simulink model "xEMU_SimulationModel3_rule1"  (R2017b)
settings: Solver=ode4  StartTime=0.0  StopTime=8192  FixedStep=0.01  RelTol=1e-3
undefined symbols (not defined in the file): a1, a2, a3, a4, ACO, BAT, Battery, DCT, DRT, EMS, ENV, Fahrzyklus_VS_modell, height_BAT, leistung, lib_bat, Maximum, Maximum_position, Num_cells, P_FC_max_long, P_FC_min_long, P_FC_step_max, Pbat_charge_max, Pbat_discharge_max, Pfc_max, Pfc_min, SOC_tar, time_peaks, TRM, velocity_peaks
libraries: simulink x5
(part 1 of 15)
settings Model: SimulationMode=accelerator  Creator=tne  LastModifiedBy=chenzhu1
settings SolverCC: ZeroCrossAlgorithm=Adaptive
settings OptimizationCC: EfficientMapNaN2IntZero=off
settings HardwareCC: TargetBitPerLong=64  TargetBitPerPointer=64  TargetBitPerSizeT=64  TargetBitPerPtrDiffT=64  TargetLongLongMode=on  TargetIntDivRoundTo=Zero  TargetEndianess=LittleEndian  TargetWordSize=64  TargetHWDeviceType=MATLAB Host  ProdEqTarget=off
settings CodeAppCC: MaxIdLength=128
settings GRTTargetCC: TargetLangStandard=C89/C90 (ANSI)  CombineOutputUpdateFcns=off  GRTInterface=on

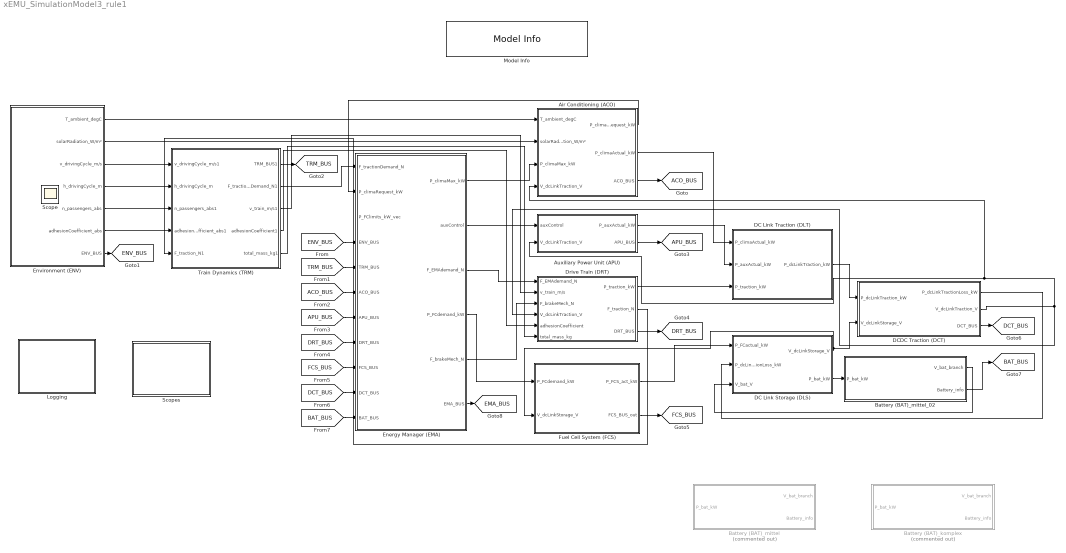
== system xEMU_SimulationModel3_rule1 ==
  Air Conditioning (ACO) : Subsystem
  Auxiliary Power Unit (APU) : Subsystem
  Battery (BAT)_komplex : Subsystem  Commented=on  AncestorBlock=lib_bat/Battery (BAT)  mask{n_series=BAT.model.n_series, n_parallel=BAT.model.n_parallel, Temp=BAT.model.Temp, SoC=BAT.model.SoC, Rser=BAT.model.Rser, R1=BAT.model.R1, Tau1=BAT.model.Tau1, R2=BAT.model.R2, Tau2=BAT.model.Tau2, Phi2=BAT.model.Phi2, R3=BAT.model.R3, Tau3=BAT.model.Tau3, Phi3=BAT.model.Phi3, R4=BAT.model.R4, Tau4=BAT.model.Tau4, R5=BAT.model.R5, Tau5=BAT.model.Tau5, Sigma2=BAT.model.Sigma2, CLim2=BAT.model.CLim2, Sigma3=BAT.model.Sigma3, CLim3=BAT.model.CLim3, ROCV=BAT.model.ROCV, UOCV=BAT.model.UOCV, OCV2=BAT.model.OCV2, SOC2=BAT.model.SOC2, TEMP2=BAT.model.TEMP2}
  Battery (BAT)_mittel : Subsystem  Commented=on  AncestorBlock=lib_bat/Battery (BAT)  mask{n_series=BAT.model.n_series, n_parallel=BAT.model.n_parallel, Temp=BAT.model.Temp, SoC=BAT.model.SoC, Rser=BAT.model.Rser, R1=BAT.model.R1, Tau1=BAT.model.Tau1, R2=BAT.model.R2, Tau2=BAT.model.Tau2, Phi2=BAT.model.Phi2, R3=BAT.model.R3, Tau3=BAT.model.Tau3, Phi3=BAT.model.Phi3, R4=BAT.model.R4, Tau4=BAT.model.Tau4, R5=BAT.model.R5, Tau5=BAT.model.Tau5, Sigma2=BAT.model.Sigma2, CLim2=BAT.model.CLim2, Sigma3=BAT.model.Sigma3, CLim3=BAT.model.CLim3, ROCV=BAT.model.ROCV, UOCV=BAT.model.UOCV, OCV2=BAT.model.OCV2, SOC2=BAT.model.SOC2, TEMP2=BAT.model.TEMP2}
  Battery (BAT)_mittel_02 : Subsystem  AncestorBlock=lib_bat/Battery (BAT)  mask{n_series=BAT.model.n_series, n_parallel=BAT.model.n_parallel, Temp=BAT.model.Temp, SoC=BAT.model.SoC, Rser=BAT.model.Rser, R1=BAT.model.R1, Tau1=BAT.model.Tau1, R2=BAT.model.R2, Tau2=BAT.model.Tau2, Phi2=BAT.model.Phi2, R3=BAT.model.R3, Tau3=BAT.model.Tau3, Phi3=BAT.model.Phi3, R4=BAT.model.R4, Tau4=BAT.model.Tau4, R5=BAT.model.R5, Tau5=BAT.model.Tau5, Sigma2=BAT.model.Sigma2, CLim2=BAT.model.CLim2, Sigma3=BAT.model.Sigma3, CLim3=BAT.model.CLim3, ROCV=BAT.model.ROCV, UOCV=BAT.model.UOCV, OCV2=BAT.model.OCV2, SOC2=BAT.model.SOC2, TEMP2=BAT.model.TEMP2}
  DC Link Storage (DLS) : Subsystem
  DC Link Traction (DLT) : Subsystem
  DCDC Traction (DCT) : Subsystem  AncestorBlock=lib_dct/DCDC Traction (DCT)  mask{fs_DCDC_Hz=DCT.fs_DCDC_Hz}
  Drive Train (DRT) : Subsystem  AncestorBlock=lib_drt/Drive Train (DRT)  mask{gearratio_drt=DRT.motor.gearratio_drt, R_wheel_drt_m=DRT.slipmodel.R_wheel_drt_m, g_drt=DRT.slipmodel.g_drt, fr_drt_abs=DRT.slipmodel.fr_drt_abs, J_drt=DRT.slipmodel.J_drt, Schub_drt=DRT.slipmodel.Schub_drt, a_drt=DRT.slipmodel.a_drt, b_drt=DRT.slipmodel.b_drt, C11_drt=DRT.slipmodel.C11_drt, speedvector=DRT.motor.speedvector, torquevector=DRT.motor.torquevector, eta=DRT.motor.eta, cosphi=DRT.motor.cosphi, I_strang=DRT.motor.I_strang, U_LL=DRT.motor.U_LL, Pv_motor=DRT.motor.Pv_motor, torque_untergrenze=DRT.motor.torque_untergrenze, torque_obergrenze=DRT.motor.torque_obergrenze, torquevector2=DRT.motor.torquevector2, speedvector2=DRT.motor.speedvector2, cosphi2=DRT.motor.cosphi2, Pv_untergrenze=DRT.motor.Pv_untergrenze, Pv_obergrenze=DRT.motor.Pv_obergrenze, U_LL_untergrenze=DRT.motor.U_LL_untergrenze, U_LL_obergrenze=DRT.motor.U_LL_obergrenze, I_strang_untergrenze=DRT.motor.I_strang_untergrenze, cosphi_obergrenze=DRT.motor.cosphi_obergrenze, cosphi_untergrenze=DRT.motor.cosphi_untergrenze, I_strang_obergrenze=DRT.motor.I_strang_obergrenze}
  Energy Manager (EMA) : Subsystem  AncestorBlock=lib_ems/Energy Manager (EMA)
  Environment (ENV) : Subsystem
  Fuel Cell System (FCS) : Subsystem  AncestorBlock=lib_fcs/Fuel Cell System (FCS)
  Logging : Subsystem
  Model Info : simulink/Model-Wide Utilities/Model Info  Frame=on  DisplayStringWithTags=|  HorizontalTextAlignment=Center  LeftAlignmentValue=0.5
      | Model name: %<ModelName>
      | Created: %<Created>
      | Model version:%<ModelVersion>
      | Last modified by: hp
      | Last modification date: %<LastModificationDate>
  Scopes : Subsystem
  Train Dynamics (TRM) : Subsystem  AncestorBlock=lib_trm/Train Dynamics (TDN)1  mask{m_train_tdn_kg=TRM.m_train_tdn_kg, Cw_tdn_abs=TRM.Cw_tdn_abs, A_tdn_m2=TRM.A_tdn_m2, e_tdn_abs=TRM.e_tdn_abs, PI_tdn=TRM.PI_tdn, m_passenger_tdn_kg=TRM.m_passenger_tdn_kg, g_drt=TRM.g_drt, gearratio_drt=DRT.motor.gearratio_drt, R_wheel_drt_m=DRT.slipmodel.R_wheel_drt_m, speedvector=DRT.motor.speedvector, torquevector=DRT.motor.torquevector, torque_untergrenze=DRT.motor.torque_untergrenze, torque_obergrenze=DRT.motor.torque_obergrenze}
  Scope : Scope
  tag scope: ACO_BUS=global, APU_BUS=global, BAT_BUS=global, DCT_BUS=global, DRT_BUS=global, EMA_BUS=global, ENV_BUS=global, FCS_BUS=global, TRM_BUS=global
  wires:
  Environment (ENV)/1(T_ambient_degC) -> Air Conditioning (ACO)/1(T_ambient_degC)
  Environment (ENV)/2(solarRadiation_W/m²) -> Air Conditioning (ACO)/2(solarRadiation_W/m²)
  Air Conditioning (ACO)/2(P_climaActual_kW) -> DC Link Traction (DLT)/1(P_climaActual_kW)
  Auxiliary Power Unit (APU)/1(P_auxActual_kW) -> DC Link Traction (DLT)/2(P_auxActual_kW)
  Environment (ENV)/7(ENV_BUS) -> [ENV_BUS]
  DC Link Storage (DLS)/1(V_dcLinkStorage_V) -> DCDC Traction (DCT)/2(V_dcLinkStorage_V), Fuel Cell System (FCS)/2(V_dcLinkStorage_V)
  DC Link Traction (DLT)/1(P_dcLinkTraction_kW) -> DCDC Traction (DCT)/1(P_dcLinkTraction_kW)
  DCDC Traction (DCT)/1(P_dcLinkTractionLoss_kW) -> DC Link Storage (DLS)/2(P_dcLinkTractionLoss_kW)
  Drive Train (DRT)/1(P_traction_kW) -> DC Link Traction (DLT)/3(P_traction_kW)
  Drive Train (DRT)/2(F_traction_N) -> Train Dynamics (TRM)/5(F_traction_N1)
  Environment (ENV)/4(h_drivingCycle_m) -> Train Dynamics (TRM)/2(h_drivingCycle_m)
  Train Dynamics (TRM)/3(v_train_m/s1) -> Drive Train (DRT)/2(v_train_m/s)
  Train Dynamics (TRM)/4(adhesionCoefficient1) -> Drive Train (DRT)/5("adhesionCoefficient ")
  Train Dynamics (TRM)/5(total_mass_kg1) -> Drive Train (DRT)/6(total_mass_kg)
  Air Conditioning (ACO)/1(P_climaRequest_kW) -> Energy Manager (EMA)/2("P_climaRequest_kW ")
  Energy Manager (EMA)/4(P_FCdemand_kW) -> Fuel Cell System (FCS)/1(P_FCdemand_kW)
  Energy Manager (EMA)/5(F_brakeMech_N) -> Drive Train (DRT)/3(F_brakeMech_N)
  Energy Manager (EMA)/6(EMA_BUS) -> [EMA_BUS]
  [TRM_BUS] -> Energy Manager (EMA)/5(TRM_BUS)
  [ACO_BUS] -> Energy Manager (EMA)/6(ACO_BUS)
  [APU_BUS] -> Energy Manager (EMA)/7(APU_BUS)
  [DRT_BUS] -> Energy Manager (EMA)/8(DRT_BUS)
  [FCS_BUS] -> Energy Manager (EMA)/9(FCS_BUS)
  [DCT_BUS] -> Energy Manager (EMA)/10(DCT_BUS)
  [BAT_BUS] -> Energy Manager (EMA)/11(BAT_BUS)
  [ENV_BUS] -> Energy Manager (EMA)/4(ENV_BUS)
  Energy Manager (EMA)/3(F_EMAdemand_N) -> Drive Train (DRT)/1(F_EMAdemand_N)
  Energy Manager (EMA)/2(auxControl) -> Auxiliary Power Unit (APU)/1(auxControl)
  Energy Manager (EMA)/1(P_climaMax_kW) -> Air Conditioning (ACO)/3(P_climaMax_kW)
  DCDC Traction (DCT)/2(V_dcLinkTraction_V) -> Drive Train (DRT)/4(V_dcLinkTraction_V), Auxiliary Power Unit (APU)/2(V_dcLinkTraction_V), Air Conditioning (ACO)/4(V_dcLinkTraction_V)
  DCDC Traction (DCT)/3(DCT_BUS) -> [DCT_BUS]
  Drive Train (DRT)/3(DRT_BUS) -> [DRT_BUS]
  Auxiliary Power Unit (APU)/2(APU_BUS) -> [APU_BUS]
  Air Conditioning (ACO)/3(ACO_BUS) -> [ACO_BUS]
  Environment (ENV)/3(v_drivingCycle_m/s) -> Train Dynamics (TRM)/1(v_drivingCycle_m/s1)
  Environment (ENV)/5(n_passengers_abs) -> Train Dynamics (TRM)/3(n_passengers_abs1)
  Environment (ENV)/6(adhesionCoefficient_abs) -> Train Dynamics (TRM)/4(adhesionCoefficient_abs1)
  Train Dynamics (TRM)/1(TRM_BUS1) -> [TRM_BUS]
  Train Dynamics (TRM)/2(F_tractionDemand_N1) -> Energy Manager (EMA)/1(F_tractionDemand_N)
  Fuel Cell System (FCS)/1(P_FCS_act_kW) -> DC Link Storage (DLS)/1(P_FCactual_kW)
  Fuel Cell System (FCS)/2(FCS_BUS_out) -> [FCS_BUS]
  DC Link Storage (DLS)/2(P_bat_kW) -> Battery (BAT)_mittel_02/1(P_bat_kW)
  Battery (BAT)_mittel_02/1(V_bat_branch) -> DC Link Storage (DLS)/3(V_bat_V)
  Battery (BAT)_mittel_02/2(Battery_info) -> [BAT_BUS]

== system xEMU_SimulationModel3_rule1/Air Conditioning (ACO) ==
  T_ambient_degC : Inport
  solarRadiation_W/m² : Inport  Port=2
  P_climaMax_kW : Inport  Port=3
  V_dcLinkTraction_V : Inport  Port=4
  Bus Creator1 : BusCreator  Inputs=3
  Constant : Constant
  Constant1 : Constant
  Divide : Product  Inputs=*/
  Divide1 : Product  Inputs=*/
  Gain : Gain  Gain=ACO.Awin/2
  Gain1 : Gain  Gain=ACO.Awall
  Gain2 : Gain  Gain=ACO.Awin
  Gain3 : Gain  Gain=116.3
  Heat gain : Fcn  Expr=u^2/ACO.R_warm
  Subtract : Sum
  Subtract1 : Sum  Inputs=+++++
  Sum : Sum  Inputs=-+|
  Tsoll : Constant  Value=25
  Unit Delay : UnitDelay  SampleTime=-1
  Wall-Conduct-Convection-Coefficient : Fcn  Expr=1/ACO.a1+ACO.s1/ACO.lambda1+ACO.s2/ACO.lambda2+ACO.s3/ACO.lambda3+1/u
  "Window-Conduct-Convection-Coeffcient " : Fcn  Expr=1/ACO.a1+ACO.swin/ACO.lambdawin+1/u
  approximation from passenger to ventilation : Gain  Gain=5/3
  efficient : Gain  Gain=1/3
  exterior coefficient : Fcn  Expr=9+3.5*u^0.66
  w-kw : Gain  Gain=1/1000
  P_climaRequest_kW : Outport
  P_climaActual_kW : Outport  Port=2
  ACO_BUS : Outport  Port=3
  wires:
  Unit Delay/1 -> ACO_BUS/1
  Gain/1 -> Subtract1/2  "Radiation"
  T_ambient_degC/1 -> Sum/2
  Tsoll/1 -> Sum/1
  Sum/1 -> Divide1/1, Divide/1
  "Window-Conduct-Convection-Coeffcient "/1 -> Divide1/2
  Wall-Conduct-Convection-Coefficient/1 -> Divide/2
  Divide/1 -> Gain1/1
  Divide1/1 -> Gain2/1
  Gain1/1 -> Subtract/1
  Gain2/1 -> Subtract/2
  Subtract/1 -> Subtract1/1  "Conduction&Convection"
  exterior coefficient/1 -> "Window-Conduct-Convection-Coeffcient "/1, Wall-Conduct-Convection-Coefficient/1
  [v_ist] -> exterior coefficient/1
  Gain3/1 -> approximation from passenger to ventilation/1, Subtract1/3  "passengers'load"
  approximation from passenger to ventilation/1 -> Subtract1/4  "ventilation"
  Subtract1/1 -> w-kw/1
  efficient/1 -> P_climaActual_kW/1, P_climaRequest_kW/1
  V_dcLinkTraction_V/1 -> Heat gain/1
  Heat gain/1 -> Subtract1/5
  w-kw/1 -> efficient/1
  Bus Creator1/1 -> Unit Delay/1
  Constant1/1 -> Bus Creator1/2  "signal2"
  Constant/1 -> Bus Creator1/1  "signal1"
  P_climaMax_kW/1 -> Bus Creator1/3  "P_Klima"
  solarRadiation_W/m²/1 -> Gain/1
  [n_passengers] -> Gain3/1

== system xEMU_SimulationModel3_rule1/Auxiliary Power Unit (APU) ==
  auxControl : Inport
  V_dcLinkTraction_V : Inport  Port=2
  Constant : Constant  Value=30
  Unit Delay : UnitDelay  SampleTime=-1
  P_auxActual_kW : Outport
  APU_BUS : Outport  Port=2
  wires:
  Constant/1 -> Unit Delay/1
  Unit Delay/1 -> APU_BUS/1, P_auxActual_kW/1  "P_aux"

== system xEMU_SimulationModel3_rule1/Battery (BAT)_komplex ==
  P_bat_kW : Inport
  Bus Creator : BusCreator  Inputs=12
  Delay : Delay  DelayLength=1
  Display1 : Display
  Divide : Product  Inputs=*/
  Gain : Gain  Gain=-1
  Gain1 : Gain  Gain=1/100
  Gain2 : Gain  Gain=-1
  Integrator1 : Integrator  LimitOutput=on  LowerSaturationLimit=0
  MATLAB Function : MATLAB Function  TreatAsAtomicUnit=on
  Scope : Scope
  Scope6 : Scope
  Subsystem : Subsystem
  cell2pack : Gain  Gain=370
  kW->W : Gain  Gain=1000
  pack2cell : Gain  Gain=1/9
  V_bat_branch : Outport
  Battery_info : Outport  Port=2
  wires:
  Bus Creator/1 -> Battery_info/1
  kW->W/1 -> Divide/1
  Delay/1 -> Gain2/1, MATLAB Function/2(I_bat), pack2cell/1  "I_bat"
  P_bat_kW/1 -> Bus Creator/5, Gain/1  "P_bat"
  Divide/1 -> Delay/1  "I_Pack_A"
  cell2pack/1 -> V_bat_branch/1, Bus Creator/1, Display1/1, Divide/2  "V_bat"
  pack2cell/1 -> Subsystem/1(In2)  "I_Cell_A"
  Subsystem/1(CellVoltage) -> cell2pack/1
  Subsystem/5(SoC_Percent) -> Gain1/1, Bus Creator/8  "SOC"
  Gain/1 -> kW->W/1  "P_bat"
  MATLAB Function/1(Battery_consume_eff_rate) -> Integrator1/1
  Gain1/1 -> Scope6/1, MATLAB Function/1(SOC_i)
  Integrator1/1 -> Scope/1
  Gain2/1 -> Bus Creator/2  "I_bat"
  [T_CellElement1] -> MATLAB Function/3(Temp)

== system xEMU_SimulationModel3_rule1/Battery (BAT)_mittel ==
  note: I positive --> Charge
  note: I negative --> Discharge
  P_bat_kW : Inport
  Battery : Subsystem
  Bus : BusCreator  Inputs=6
  Bus Creator1 : BusCreator  Inputs=12
  Bus Selector : BusSelector  OutputSignals=soc.signal1
  Delay : Delay  DelayLength=1
  Display1 : Display
  Divide : Product  Inputs=*/
  Gain : Gain  Gain=-1
  Gain1 : Gain  Gain=-1
  Scope : Scope
  Scope1 : Scope
  Subsystem1 : Subsystem  Commented=on
  To Workspace : ToWorkspace  VariableName=Batt_temp_1s1p_thevenin  SaveFormat=Structure With Time  SampleTime=-1
  cell2pack : Gain  Gain=370
  cell2pack1 : Gain
  kW->W : Gain  Gain=1000
  pack2cell : Gain  Gain=1/9
  V_bat_branch : Outport
  Battery_info : Outport  Port=2
  wires:
  kW->W/1 -> Divide/1
  Delay/1 -> Gain1/1, pack2cell/1
  P_bat_kW/1 -> Gain/1, Bus Creator1/5  "P_bat"
  Divide/1 -> Delay/1  "I_Pack_A"
  cell2pack/1 -> V_bat_branch/1, Display1/1, Divide/2, Bus Creator1/1  "V_bat"
  pack2cell/1 -> Battery/1(I_Bat_source[A])  "I_Cell_A"
  Battery/3(CellVoltage) -> Bus/3, cell2pack/1, Scope1/1
  Gain/1 -> kW->W/1
  Battery/6(SoC_[0..1]) -> Bus/6
  Battery/2(CellPower) -> Bus/2
  Battery/5(CellTemp) -> To Workspace/1, Scope/1, Bus/5
  Battery/4(CellVoltage1) -> Bus/4
  Battery/1(SoC_Percent) -> Bus/1  "soc"
  Bus/1 -> Bus Selector/1
  Bus Selector/1 -> cell2pack1/1  "<signal1>"
  Bus Creator1/1 -> Battery_info/1
  cell2pack1/1 -> Bus Creator1/8  "SOC"
  Gain1/1 -> Bus Creator1/9  "I_bat"

== system xEMU_SimulationModel3_rule1/Battery (BAT)_mittel_02 ==
  note: I positive --> Charge
  note: I negative --> Discharge
  P_bat_kW : Inport
  " " : Gain
  Bus : BusCreator  Inputs=6
  Bus Creator1 : BusCreator  Inputs=12
  Bus Selector : BusSelector  OutputSignals=soc
  Cell : Subsystem
  Cell_temperatur : Scope
  Delay : Delay  DelayLength=1
  Display1 : Display
  Divide : Product  Inputs=*/
  Gain : Gain  Gain=-1
  Gain1 : Gain  Gain=-1
  Scope1 : Scope
  Soc in % : Display
  To Workspace : ToWorkspace  VariableName=Batt_temp_1s1p_thevenin  SaveFormat=Structure With Time  SampleTime=-1
  cell2pack : Gain  Gain=370
  cell_voltage : Display
  kW->W : Gain  Gain=1000
  pack2cell : Gain  Gain=1/9
  V_bat_branch : Outport
  Battery_info : Outport  Port=2
  wires:
  kW->W/1 -> Divide/1
  Delay/1 -> Gain1/1, pack2cell/1
  P_bat_kW/1 -> Gain/1, Bus Creator1/5  "P_bat"
  Divide/1 -> Delay/1  "I_Pack_A"
  cell2pack/1 -> V_bat_branch/1, Display1/1, Divide/2, Bus Creator1/1  "V_bat"
  pack2cell/1 -> Cell/1(ExcitationCurrent)  "I_Cell_A"
  Cell/5(TotalVoltage) -> cell2pack/1, Scope1/1, Bus/3, cell_voltage/1  "cell_voltage"
  Gain/1 -> kW->W/1
  Cell/9(TemperatureVector) -> Bus/6, Cell_temperatur/1, To Workspace/1  "cell_temperature"
  Cell/6(TotalCurrent) -> Bus/4  "cell_current"
  Cell/4(SocVector) -> Soc in %/1, Bus/1  "soc"
  Bus Selector/1 -> " "/1  "<soc>"
  Bus Creator1/1 -> Battery_info/1
  " "/1 -> Bus Creator1/8  "SOC"
  Gain1/1 -> Bus Creator1/9  "I_bat"
  Cell/2(CurrentVector) -> ?
  Bus/1 -> Bus Selector/1
  Cell/7(TotalHeatGeneration) -> Bus/5  "cell_heat"

== system xEMU_SimulationModel3_rule1/DC Link Storage (DLS) ==
  note: die Summe aller Leistung und Verluste
  note: die Versorgung aus FC
  note: die Versorgung aus Battery
  P_FCactual_kW : Inport
  P_dcLinkTractionLoss_kW : Inport  Port=2
  V_bat_V : Inport  Port=3
  Constant : Constant
  Integrator1 : Integrator
  Integrator2 : Integrator
  MATLAB Function : MATLAB Function  TreatAsAtomicUnit=on
  Subtract : Sum  Inputs=-+
  V_dcLinkStorage_V : Outport
  P_bat_kW : Outport  Port=2
  tag scope: P_Demand=global
  wires:
  V_bat_V/1 -> Integrator2/1, V_dcLinkStorage_V/1
  Subtract/1 -> P_bat_kW/1
  P_FCactual_kW/1 -> Subtract/1
  P_dcLinkTractionLoss_kW/1 -> [P_Demand], Subtract/2
  Constant/1 -> Integrator1/1
  Integrator1/1 -> MATLAB Function/1(t)
  Integrator2/1 -> MATLAB Function/2(v_bat_total)
  MATLAB Function/1(v_bat_average) -> ?

== system xEMU_SimulationModel3_rule1/DC Link Traction (DLT) ==
  P_climaActual_kW : Inport
  P_auxActual_kW : Inport  Port=2
  P_traction_kW : Inport  Port=3
  Sum : Sum  Inputs=|+++
  P_dcLinkTraction_kW : Outport
  wires:
  P_auxActual_kW/1 -> Sum/2
  P_climaActual_kW/1 -> Sum/1
  P_traction_kW/1 -> Sum/3
  Sum/1 -> P_dcLinkTraction_kW/1

== system xEMU_SimulationModel3_rule1/DCDC Traction (DCT) ==
  P_dcLinkTraction_kW : Inport
  V_dcLinkStorage_V : Inport  Port=2
  DCDC_elektrisch_Modellierung : Subsystem
  DCDC_thermische_Modellirung : Subsystem
  P_dcLinkTractionLoss_kW : Outport
  V_dcLinkTraction_V : Outport  Port=2
  DCT_BUS : Outport  Port=3
  wires:
  P_dcLinkTraction_kW/1 -> DCDC_elektrisch_Modellierung/1(P_load_vor_dcdc_converter1)  "P_load_vor_dcdc_converter"
  V_dcLinkStorage_V/1 -> DCDC_elektrisch_Modellierung/2(V_dcLinkStorage_V1)
  DCDC_elektrisch_Modellierung/1(V_dcLinkTraction_V) -> V_dcLinkTraction_V/1
  DCDC_elektrisch_Modellierung/4("IGBT_Pv_kW ") -> DCDC_thermische_Modellirung/2(igbt_loss_kW)
  DCDC_elektrisch_Modellierung/2("DCT_BUS ") -> DCT_BUS/1
  DCDC_elektrisch_Modellierung/5(Diode_Pv_kW) -> DCDC_thermische_Modellirung/1(Diode_loss_kW)
  DCDC_thermische_Modellirung/1(IGBT_Temp_Celsius) -> DCDC_elektrisch_Modellierung/4(IGBT _Junction_Temp1)
  DCDC_thermische_Modellirung/2(Diode_Temp_Celsius) -> DCDC_elektrisch_Modellierung/3(Diode _Junction_Temp1)
  DCDC_elektrisch_Modellierung/3(P_dcLinkTractionLoad_kW) -> P_dcLinkTractionLoss_kW/1

== system xEMU_SimulationModel3_rule1/Drive Train (DRT) ==
  F_EMAdemand_N : Inport
  v_train_m/s : Inport  Port=2
  F_brakeMech_N : Inport  Port=3
  V_dcLinkTraction_V : Inport  Port=4
  "adhesionCoefficient " : Inport  Port=5
  total_mass_kg : Inport  Port=6
  Aufteilung rad-undmotormomente : Subsystem
  Bus Creator : BusCreator  Inputs=5
  Converter and traction motor : Subsystem
  Gain : Gain  Gain=gearratio_drt
  Mechanical Brake : Subsystem
  Product{,1..4} (5 alike) : Product
  "Slipmodel and Traction " : Subsystem
  Subtract : Sum
  Sum : Sum  Inputs=++|
  Unit Delay : UnitDelay  SampleTime=-1
  gear efficiency : MATLAB Function  TreatAsAtomicUnit=on
  gear_efficiency : Constant  Value=DRT.motor.gear_efficiency_drt
  P_traction_kW : Outport
  F_traction_N : Outport  Port=2
  DRT_BUS : Outport  Port=3
  wires:
  Unit Delay/1 -> DRT_BUS/1
  V_dcLinkTraction_V/1 -> Converter and traction motor/3(v_dc)
  F_EMAdemand_N/1 -> Aufteilung rad-undmotormomente/1(F_EMAdemand_N)
  Mechanical Brake/1(Out1) -> Sum/1
  Product/1 -> P_traction_kW/1  "P_motor_elekrisch+Pacdc"
  Converter and traction motor/1("T_singelmotor_Nm ") -> Gain/1  "m"
  Aufteilung rad-undmotormomente/4(T_brake_axis_Nm) -> Mechanical Brake/1(In1)
  Gain/1 -> gear efficiency/1(t_motor)
  Aufteilung rad-undmotormomente/1(T_demandperdrive_Nm) -> Converter and traction motor/1(T_demand)
  Aufteilung rad-undmotormomente/2(n_motor_rpm) -> Converter and traction motor/2(n), Bus Creator/5  "n_motor_rpm"
  F_brakeMech_N/1 -> Aufteilung rad-undmotormomente/2(F_brake_N)
  Converter and traction motor/2("Pel_singlemotor_kW ") -> Product/2
  "Slipmodel and Traction "/2(WheelSpeed_rad/s) -> Aufteilung rad-undmotormomente/3("WheelSpeed_rad/s ")
  Sum/1 -> "Slipmodel and Traction "/1(T_EMAdemandper_axis_Nm)
  "adhesionCoefficient "/1 -> "Slipmodel and Traction "/3(adhesionCoefficient_abs)
  total_mass_kg/1 -> "Slipmodel and Traction "/4(total mass_kg)
  v_train_m/s/1 -> "Slipmodel and Traction "/2(v_train_m/s)
  Bus Creator/1 -> Unit Delay/1
  "Slipmodel and Traction "/1(F_traction_peraxis_N) -> Product2/2
  Product2/1 -> F_traction_N/1
  Product3/1 -> Bus Creator/2  "P_motor_mechanisch"
  Aufteilung rad-undmotormomente/3(Number_drives_available) -> Product/1, Product1/1, Product4/1, Product3/1, Product2/1, "Slipmodel and Traction "/5(numberdrivesavailable)
  [P_motor_mechanic] -> Product3/2  "P_motor_mechanic"
  [Pv_motor] -> Product4/2
  Product4/1 -> Subtract/2, Bus Creator/3  "P_motor_Verlust"
  Product1/1 -> Subtract/1, Bus Creator/1  "P_acdc_Verlust"
  Subtract/1 -> Bus Creator/4  "P_motor_Verlust+Pacdc"
  [Pv_ACDC] -> Product1/2  "P_acdc_Verlust"
  gear efficiency/1(t_axis) -> Sum/2
  gear_efficiency/1 -> gear efficiency/2(data)

== system xEMU_SimulationModel3_rule1/Energy Manager (EMA) ==
  F_tractionDemand_N : Inport
  "P_climaRequest_kW " : Inport  Port=2
  P_FClimits_kW_vec : Inport  Port=3
  ENV_BUS : Inport  Port=4
  TRM_BUS : Inport  Port=5
  ACO_BUS : Inport  Port=6
  APU_BUS : Inport  Port=7
  DRT_BUS : Inport  Port=8
  FCS_BUS : Inport  Port=9
  DCT_BUS : Inport  Port=10
  BAT_BUS : Inport  Port=11
  Berechnung der available Traktionsleitung : Subsystem
  Bus Creator1 : BusCreator  Inputs=8
  Bus Selector : BusSelector  OutputSignals=v_drivingCycle_m/s,Steigung%
  Bus Selector1 : BusSelector  OutputSignals=v_train_m/s
  Bus Selector2 : BusSelector  OutputSignals=P_motor_Verlust+Pacdc,n_motor_rpm
  Bus Selector3 : BusSelector  OutputSignals=P_dcdc_Verlust,P_dcLinkTractionLoad
  Bus Selector4 : BusSelector  OutputSignals=SOC,V_bat
  Demux : Demux
  Display{,1..3} (4 alike) : Display
  Kern von EMS : Subsystem
  Scope : Scope
  Umrechnung von Kraft zu Leistung : Subsystem
  Umrechnung von Leistung auf Kraft : Subsystem
  Umrechnung von Leistung auf Kraft2 : Subsystem
  P_climaMax_kW : Outport
  auxControl : Outport  Port=2
  F_EMAdemand_N : Outport  Port=3
  P_FCdemand_kW : Outport  Port=4
  F_brakeMech_N : Outport  Port=5
  EMA_BUS : Outport  Port=6
  tag scope: F_EMAdemand_N=global, P_apu=global, P_clima=global, n_motor_rpm=global, v_soll=global
  wires:
  Bus Selector/1 -> Kern von EMS/2(<v_train_m/s>_soll), [v_soll]  "<v_drivingCycle_m/s>"
  Bus Selector1/1 -> Umrechnung von Kraft zu Leistung/2(<v_train_m/s>), Umrechnung von Leistung auf Kraft2/3(<v_train_m/s>), Umrechnung von Leistung auf Kraft/3(<v_drivingCycle_m/s>)  "<v_train_m/s>"
  Kern von EMS/1(P_FCdemand_kW) -> P_FCdemand_kW/1, Bus Creator1/6  "P_Fc_demand"
  [mode] -> Bus Creator1/7  "mode"
  [P_apu] -> Bus Creator1/4  "P_apu"
  [P_clima] -> Bus Creator1/3  "P_clima"
  Bus Selector3/1 -> Berechnung der available Traktionsleitung/3(<P_dcdc_Verlust>), Umrechnung von Kraft zu Leistung/4(<P_dcdc_Verlust>)  "<P_dcdc_Verlust>"
  Bus Selector2/1 -> Berechnung der available Traktionsleitung/2(<P_motor_Verlust+Pacdc>), Umrechnung von Kraft zu Leistung/3(<P_motor_Verlust+Pacdc>)  "<P_motor_Verlust+Pacdc>"
  Bus Creator1/1 -> EMA_BUS/1
  Bus Selector4/2 -> Kern von EMS/4(<V_bat_V>)  "<V_bat>"
  Bus Selector4/1 -> Kern von EMS/3(<SOC_perc>)  "<SOC>"
  APU_BUS/1 -> [P_apu]
  ENV_BUS/1 -> Bus Selector/1
  TRM_BUS/1 -> Bus Selector1/1
  DRT_BUS/1 -> Bus Selector2/1
  BAT_BUS/1 -> Bus Selector4/1
  "P_climaRequest_kW "/1 -> P_climaMax_kW/1, [P_clima]
  DCT_BUS/1 -> Bus Selector3/1
  P_FClimits_kW_vec/1 -> Demux/1
  Bus Selector2/2 -> [n_motor_rpm]  "<n_motor_rpm>"
  Umrechnung von Kraft zu Leistung/2(P_drive_demand) -> Umrechnung von Leistung auf Kraft/2(P_drive_demand), Bus Creator1/1
  F_tractionDemand_N/1 -> Umrechnung von Kraft zu Leistung/1(F_tractionDemand_N)
  Umrechnung von Kraft zu Leistung/1(P_load_wunsch) -> Display/1, Kern von EMS/1(P_load_wunsch_kw)
  Kern von EMS/2(P_load_available) -> Display1/1, Scope/1, Berechnung der available Traktionsleitung/1(P_load_available)
  Berechnung der available Traktionsleitung/1(P_traction_available) -> Display2/1, Umrechnung von Leistung auf Kraft/1(P_traction_available)
  Umrechnung von Leistung auf Kraft2/3(F_EMAdemand_N) -> Display3/1, [F_EMAdemand_N], F_EMAdemand_N/1
  Umrechnung von Leistung auf Kraft/1(F_brakeMech_N) -> Umrechnung von Leistung auf Kraft2/1(F_brakeMech_N1)
  Umrechnung von Leistung auf Kraft/2(F_EMAdemand_N) -> Umrechnung von Leistung auf Kraft2/2(F_EMAdemand_N1)
  Umrechnung von Leistung auf Kraft2/1(F_available_nach_EMA) -> Bus Creator1/8
  Umrechnung von Leistung auf Kraft2/2(F_brakeMech_N) -> F_brakeMech_N/1

== system xEMU_SimulationModel3_rule1/Environment (ENV) ==
  %-1 : Gain  Gain=1/100
  1-D Lookup Table : Lookup_n-D  NumberOfTableDimensions=1  BreakpointsForDimension1=ENV.height.position  Table=ENV.height.Height  InternalRulePriority=Speed  RndMeth=Simplest  InputSameDT=on
  Bus Creator : BusCreator  Inputs=2
  Fahrzyklus : simulink/Sources/Repeating Sequence  rep_seq_t=ENV.fahrzyklus.time  rep_seq_y=ENV.fahrzyklus.v
  Integrator : Integrator
  Integrator1 : Integrator
  Scope1 : Scope
  Steigung : Lookup_n-D  NumberOfTableDimensions=1  BreakpointsForDimension1=ENV.steigung.position  Table=ENV.steigung.Steigung  InternalRulePriority=Speed  RndMeth=Simplest  InputSameDT=on
  T_ambient : Constant  Value=ENV.temperatur
  adhesionCoefficient : Constant  Value=ENV.adhesionCoefficient
  number of Passengers : Constant  Value=ENV.number_passengers
  solarRadiation : Constant  Value=ENV.solarRadiation
  T_ambient_degC : Outport
  solarRadiation_W/m² : Outport  Port=2
  v_drivingCycle_m/s : Outport  Port=3
  h_drivingCycle_m : Outport  Port=4
  n_passengers_abs : Outport  Port=5
  adhesionCoefficient_abs : Outport  Port=6
  ENV_BUS : Outport  Port=7
  tag scope: n_passengers=global
  wires:
  Bus Creator/1 -> ENV_BUS/1
  Fahrzyklus/1 -> v_drivingCycle_m/s/1, Bus Creator/1, Integrator1/1  "v_drivingCycle_m/s"
  Steigung/1 -> Integrator/1, Bus Creator/2, %-1/1  "Steigung%"
  adhesionCoefficient/1 -> adhesionCoefficient_abs/1
  T_ambient/1 -> T_ambient_degC/1
  solarRadiation/1 -> solarRadiation_W/m²/1
  Integrator1/1 -> 1-D Lookup Table/1, Steigung/1
  %-1/1 -> Scope1/1, h_drivingCycle_m/1
  number of Passengers/1 -> [n_passengers], n_passengers_abs/1
  Integrator/1 -> ?

== system xEMU_SimulationModel3_rule1/Fuel Cell System (FCS) ==
  P_FCdemand_kW : Inport
  V_dcLinkStorage_V : Inport  Port=2
  "FC_DCDC " : Subsystem  AncestorBlock=lib_fcs/Fuel Cell System (FCS)/FC_controller
  "FC_controller " : Subsystem
  FC_system : Subsystem  AncestorBlock=lib_fcs/Fuel Cell System (FCS)/FC_controller
  Unit Delay : UnitDelay  SampleTime=-1
  P_FCS_act_kW : Outport
  FCS_BUS_out : Outport  Port=2
  wires:
  Unit Delay/1 -> FCS_BUS_out/1
  FC_system/1(FCS_state_BUS) -> "FC_controller "/3(FC_state_BUS)
  "FC_DCDC "/1(P_DCDC_act_kW) -> P_FCS_act_kW/1, "FC_controller "/5(p_fc_act)
  FC_system/3(i_act_fcs) -> "FC_DCDC "/4(i_act_fcs)
  "FC_DCDC "/2(i_demand_dcdc_fc) -> FC_system/2(i_demand_dcdc_fc)
  "FC_controller "/2(i_demand) -> "FC_DCDC "/1(i_demand_ext)
  FC_system/2(V_FCS) -> "FC_DCDC "/3(V_FCS), "FC_controller "/4(V_FCS)
  "FC_controller "/1(FCS_BUS) -> Unit Delay/1
  V_dcLinkStorage_V/1 -> "FC_controller "/2(V_dcLink), "FC_DCDC "/2(V_dcLink)
  P_FCdemand_kW/1 -> FC_system/1("P_fc "), "FC_controller "/1(p_demand_ext)

== system xEMU_SimulationModel3_rule1/Logging ==
  To Workspace : ToWorkspace  VariableName=bat_bus  SaveFormat=Timeseries  SampleTime=-1
  wires:
  [BAT_BUS] -> To Workspace/1

== system xEMU_SimulationModel3_rule1/Scopes ==
  Battery Scope : Subsystem
  Energy Manager Scope : Subsystem
  "Fuel cell Scope " : Subsystem
  Train Dynamics&Environment Scope : Subsystem

== system xEMU_SimulationModel3_rule1/Train Dynamics (TRM) ==
  v_drivingCycle_m/s1 : Inport
  h_drivingCycle_m : Inport  Port=2
  n_passengers_abs1 : Inport  Port=3
  adhesionCoefficient_abs1 : Inport  Port=4
  F_traction_N1 : Inport  Port=5
  Variant Subsystem : Subsystem  Variant=on  OverrideUsingVariant=Variant
  TRM_BUS1 : Outport
  F_tractionDemand_N1 : Outport  Port=2
  v_train_m/s1 : Outport  Port=3
  adhesionCoefficient1 : Outport  Port=4
  total_mass_kg1 : Outport  Port=5
  tag scope: total_mass=global, v_ist=global
  wires:
  Variant Subsystem/2(F_tractionDemand_N) -> F_tractionDemand_N1/1  "F_tractionDemand_N"
  Variant Subsystem/3(v_train_m/s) -> [v_ist], v_train_m/s1/1  "v_train_m/s"
  F_traction_N1/1 -> Variant Subsystem/5(F_traction_N)
  adhesionCoefficient_abs1/1 -> Variant Subsystem/4(adhesionCoefficient_abs)
  n_passengers_abs1/1 -> Variant Subsystem/3(n_passengers_abs)
  h_drivingCycle_m/1 -> Variant Subsystem/2(h_drivingCycle_m)
  Variant Subsystem/1(TRM_BUS) -> TRM_BUS1/1
  Variant Subsystem/4(adhesionCoefficient) -> adhesionCoefficient1/1
  Variant Subsystem/5(total_mass_kg) -> [total_mass], total_mass_kg1/1
  v_drivingCycle_m/s1/1 -> Variant Subsystem/1(v_drivingCycle_m/s)

== system xEMU_SimulationModel3_rule1/Battery (BAT)_komplex/Subsystem ==
  In2 : Inport
  ActiveBalancing : Subsystem
  ActiveBalancingCellCurrents : Constant  Value=[0]
  CellCurrentMatrices : Subsystem
  CellCurrents : Subsystem
  CellPowerValues : Subsystem
  CellVoltageMatrices : Subsystem
  Demux : Demux  Outputs=2
  ElectricalCircuit : Subsystem
  MatrixAxC : Subsystem
  MatrixX_alg : Subsystem
  PowerMatrix : Subsystem
  SystemStates : Subsystem
  Thermal : Subsystem
  CellVoltage : Outport
  CellPower : Outport  Port=2
  CellTemp : Outport  Port=3
  CellVoltage1 : Outport  Port=4
  SoC_Percent : Outport  Port=5
  tag scope: InputCurrent=global
  wires:
  ActiveBalancingCellCurrents/1 -> ActiveBalancing/1(CellCurrents)
  PowerMatrix/1(Components) -> CellPowerValues/1(CellPower)
  CellPowerValues/1(Out1) -> CellPower/1
  Thermal/1(Out1) -> CellTemp/1  "CellTemperature"
  Demux/2 -> CellVoltage1/1
  Demux/1 -> CellVoltage/1  "Cell_Voltage"
  CellCurrentMatrices/1(Components) -> CellCurrents/1(CellCurrents)
  In2/1 -> [InputCurrent]
  ElectricalCircuit/1(Out1) -> SoC_Percent/1
  CellVoltageMatrices/1(Components) -> Demux/1

== system xEMU_SimulationModel3_rule1/Battery (BAT)_mittel/Battery ==
  I_Bat_source[A] : Inport
  'ID3_ObjR : GotoTagVisibility  GotoTag=ID3_ObjR
  'ID3_ObjTau : GotoTagVisibility  GotoTag=ID3_ObjTau
  'ID4_ObjR : GotoTagVisibility  GotoTag=ID4_ObjR
  'ID4_ObjTau : GotoTagVisibility  GotoTag=ID4_ObjTau
  'ID5_ObjR : GotoTagVisibility  GotoTag=ID5_ObjR
  'ID5_ObjTau : GotoTagVisibility  GotoTag=ID5_ObjTau
  'State1 : GotoTagVisibility  GotoTag=State1
  'State2 : GotoTagVisibility  GotoTag=State2
  'State3 : GotoTagVisibility  GotoTag=State3
  'T_CellElement1 : GotoTagVisibility  GotoTag=T_CellElement1
  ActBal1 : GotoTagVisibility  GotoTag=ActBal1
  ActiveBalancing : Subsystem
  ActiveBalancingCellCurrents : Constant  Value=[0]
  BalancerBus_goto : GotoTagVisibility  GotoTag=BalancerBus
  CellCurrentMatrices : Subsystem
  CellCurrents : Subsystem
  CellPowerValues : Subsystem
  CellVoltageMatrices : Subsystem
  Demux : Demux  Outputs=2
  ElectricalCircuit : Subsystem
  ID2_ObjR : GotoTagVisibility  GotoTag=ID2_ObjR
  ID6_ObjV : GotoTagVisibility  GotoTag=ID6_ObjV
  I_CellElement_goto1 : GotoTagVisibility  GotoTag=I_CellElement1
  InputCurrent_goto : GotoTagVisibility  GotoTag=InputCurrent
  MatrixAxC : Subsystem
  MatrixX_alg : Subsystem
  P_CellElement_goto1 : GotoTagVisibility  GotoTag=P_CellElement1
  PowerMatrix : Subsystem
  SOC_fraction : Gain  Gain=0.01
  StatesBus_goto : GotoTagVisibility  GotoTag=StatesBus
  SystemStates : Subsystem
  Thermal : Subsystem
  SoC_Percent : Outport
  CellPower : Outport  Port=2
  CellVoltage : Outport  Port=3
  CellVoltage1 : Outport  Port=4
  CellTemp : Outport  Port=5
  SoC_[0..1] : Outport  Port=6
  tag scope: InputCurrent=scoped
  wires:
  Thermal/1(CellTemp_Bus) -> CellTemp/1
  ActiveBalancingCellCurrents/1 -> ActiveBalancing/1(CellCurrents)
  CellCurrentMatrices/1(Components) -> CellCurrents/1(CellCurrents)
  CellPowerValues/1(Out1) -> CellPower/1
  CellVoltageMatrices/1(Components) -> Demux/1
  PowerMatrix/1(Components) -> CellPowerValues/1(CellPower)
  I_Bat_source[A]/1 -> [InputCurrent]
  Demux/2 -> CellVoltage1/1
  Demux/1 -> CellVoltage/1
  SOC_fraction/1 -> SoC_[0..1]/1
  ElectricalCircuit/1(SoC_%_Bus) -> SoC_Percent/1, SOC_fraction/1

== system xEMU_SimulationModel3_rule1/Battery (BAT)_mittel/Subsystem1 ==
  In2 : Inport
  ActiveBalancing : Subsystem
  ActiveBalancingCellCurrents : Constant  Value=[0]
  CellCurrentMatrices : Subsystem
  CellCurrents : Subsystem
  CellPowerValues : Subsystem
  CellVoltageMatrices : Subsystem
  Demux : Demux  Outputs=2
  ElectricalCircuit : Subsystem
  MatrixAxC : Subsystem
  MatrixX_alg : Subsystem
  PowerMatrix : Subsystem
  SystemStates : Subsystem
  Thermal : Subsystem
  CellVoltage : Outport
  CellPower : Outport  Port=2
  CellTemp : Outport  Port=3
  CellVoltage1 : Outport  Port=4
  SoC_Percent : Outport  Port=5
  tag scope: InputCurrent=global
  wires:
  ActiveBalancingCellCurrents/1 -> ActiveBalancing/1(CellCurrents)
  PowerMatrix/1(Components) -> CellPowerValues/1(CellPower)
  CellPowerValues/1(Out1) -> CellPower/1
  Thermal/1(Out1) -> CellTemp/1  "CellTemperature"
  Demux/2 -> CellVoltage1/1
  Demux/1 -> CellVoltage/1  "Cell_Voltage"
  CellCurrentMatrices/1(Components) -> CellCurrents/1(CellCurrents)
  In2/1 -> [InputCurrent]
  ElectricalCircuit/1(Out1) -> SoC_Percent/1
  CellVoltageMatrices/1(Components) -> Demux/1

== system xEMU_SimulationModel3_rule1/Battery (BAT)_mittel_02/Cell ==
  ExcitationCurrent : Inport
  BalancingCurrent : Inport  Port=2
  AmbientTemperature : Inport  Port=3
  Reset : Inport  Port=4
  ActiveBalancing : Subsystem
  CellCurrentMatrices : Subsystem
  CellCurrents : Subsystem
  CellPowerValues : Subsystem
  CellVoltageMatrices : Subsystem
  ElectricalCircuit : Subsystem
  MatrixAxC : Subsystem
  MatrixX_alg : Subsystem
  NumCellElements : Constant
  PowerMatrix : Subsystem
  SoC_Vector : Subsystem
  SystemStates : Subsystem
  Temperature_Vector : Subsystem
  Thermal : Subsystem
  TotalValues : Subsystem
  VoltageVector : Outport
  CurrentVector : Outport  Port=2
  OhmicHeatGenerationVector : Outport  Port=3
  SocVector : Outport  Port=4
  TotalVoltage : Outport  Port=5
  TotalCurrent : Outport  Port=6
  TotalHeatGeneration : Outport  Port=7
  NumberOfBatteries : Outport  Port=8
  TemperatureVector : Outport  Port=9
  ProbeTemperatureVector : Outport  Port=10
  tag scope: AirTemperature=global, InputCurrent=global, Reset=global
  wires:
  Temperature_Vector/1(TemperatureVector) -> TemperatureVector/1
  BalancingCurrent/1 -> ActiveBalancing/1(CellCurrents)
  TotalValues/1(Current) -> TotalCurrent/1
  CellCurrentMatrices/1(Components) -> CellCurrents/1(CellCurrents), CurrentVector/1
  PowerMatrix/1(Components) -> OhmicHeatGenerationVector/1, CellPowerValues/1(CellPower)
  TotalValues/3(Power) -> TotalHeatGeneration/1
  TotalValues/2(Voltage) -> TotalVoltage/1
  SoC_Vector/1(SocVector) -> SocVector/1
  Reset/1 -> [Reset]
  [ThermalProbeTemperatures] -> ProbeTemperatureVector/1
  ExcitationCurrent/1 -> [InputCurrent]
  NumCellElements/1 -> NumberOfBatteries/1
  CellVoltageMatrices/1(Components) -> VoltageVector/1
  AmbientTemperature/1 -> [AirTemperature]

== system xEMU_SimulationModel3_rule1/DCDC Traction (DCT)/DCDC_elektrisch_Modellierung ==
  note: schaltverlust diode
  note: diodeverlust
  note: gesamte verluste
      | in DCDC wandler
  note: igbtverlust
  P_load_vor_dcdc_converter1 : Inport
  V_dcLinkStorage_V1 : Inport  Port=2
  Diode _Junction_Temp1 : Inport  Port=3
  IGBT _Junction_Temp1 : Inport  Port=4
  Add5 : Sum  Inputs=+++
  Add6 : Sum
  Bus Creator1 : BusCreator  Inputs=3
  Delay : Delay  DelayLength=1
  Delay1 : Delay  DelayLength=1
  Divide2 : Product  Inputs=*/
  Efficiency measurment : Subsystem
  Efficiency measurment1 : Subsystem
  Efficiency1 : Display
  Efficiency2 : Display
  Gain{1,7..9} (4 alike) : Gain  Gain=1 / 1000
  Gain2 : Gain  Gain=1 / 6
  Gain3 : Gain  Gain=1 / 6
  Gain6 : Gain  Gain=1000
  Unit Delay1 : UnitDelay  SampleTime=-1
  Zwischenkreisspanung1 : Constant  Value=DCT.dc_dink_voltage
  n-D Lookup Diode : Lookup_n-D  NumberOfTableDimensions=4  BreakpointsForDimension1=DCT.loss_diode.D1_U_B  BreakpointsForDimension2=DCT.loss_diode.D2_U_DC  BreakpointsForDimension3=DCT.loss_diode.D3_I_DC  BreakpointsForDimension4=DCT.loss_diode.D4_T_jun  Table=DCT.loss_diode.loss  InternalRulePriority=Speed  RndMeth=Simplest  InputSameDT=on
  n-D Lookup IGBT : Lookup_n-D  NumberOfTableDimensions=4  BreakpointsForDimension1=DCT.loss_igbt.D1_U_B  BreakpointsForDimension2=DCT.loss_igbt.D2_U_DC  BreakpointsForDimension3=DCT.loss_igbt.D3_I_DC  BreakpointsForDimension4=DCT.loss_igbt.D4_T_jun  Table=DCT.loss_igbt.loss  InternalRulePriority=Speed  RndMeth=Simplest  InputSameDT=on
  n-D Lookup Inductor : Lookup_n-D  NumberOfTableDimensions=4  BreakpointsForDimension1=DCT.loss_inductor.D1_U_B  BreakpointsForDimension2=DCT.loss_inductor.D2_U_DC  BreakpointsForDimension3=DCT.loss_inductor.D3_I_DC  BreakpointsForDimension4=DCT.loss_inductor.D4_T_jun  Table=DCT.loss_inductor.loss  InternalRulePriority=Speed  RndMeth=Simplest  InputSameDT=on
  V_dcLinkTraction_V : Outport
  "DCT_BUS " : Outport  Port=2
  P_dcLinkTractionLoad_kW : Outport  Port=3
  "IGBT_Pv_kW " : Outport  Port=4
  Diode_Pv_kW : Outport  Port=5
  tag scope: Loss_Inductor=global
  wires:
  Gain8/1 -> Delay1/1
  V_dcLinkStorage_V1/1 -> n-D Lookup IGBT/1, n-D Lookup Diode/1, n-D Lookup Inductor/1
  Gain6/1 -> Divide2/1
  Divide2/1 -> n-D Lookup Diode/3, n-D Lookup Inductor/3, n-D Lookup IGBT/3
  Gain7/1 -> Efficiency measurment1/2(In2), Bus Creator1/1, Add6/2  "P_dcdc_Verlust"
  Add5/1 -> Gain7/1
  Bus Creator1/1 -> Unit Delay1/1
  Add6/1 -> P_dcLinkTractionLoad_kW/1, Efficiency measurment/2(In2), Bus Creator1/2  "P_dcLinkTractionLoad"
  n-D Lookup IGBT/1 -> Gain2/1, Add5/1
  Diode _Junction_Temp1/1 -> n-D Lookup Inductor/4, n-D Lookup IGBT/4
  Unit Delay1/1 -> "DCT_BUS "/1
  Gain9/1 -> Delay/1
  IGBT _Junction_Temp1/1 -> n-D Lookup Diode/4
  n-D Lookup Diode/1 -> Add5/2, Gain3/1
  Zwischenkreisspanung1/1 -> V_dcLinkTraction_V/1, n-D Lookup Diode/2, Divide2/2, n-D Lookup Inductor/2, n-D Lookup IGBT/2
  n-D Lookup Inductor/1 -> Gain1/1
  Gain1/1 -> [Loss_Inductor], Add5/3
  Gain2/1 -> Gain8/1
  Gain3/1 -> Gain9/1
  Efficiency measurment1/1(Efficiency) -> Efficiency2/1
  Efficiency measurment/1(Efficiency) -> Efficiency1/1
  P_load_vor_dcdc_converter1/1 -> Efficiency measurment/1(In1), Efficiency measurment1/1(In1), Add6/1, Bus Creator1/3, Gain6/1  "P_load_vor_dcdc_converter"
  Delay1/1 -> "IGBT_Pv_kW "/1
  Delay/1 -> Diode_Pv_kW/1

== system xEMU_SimulationModel3_rule1/DCDC Traction (DCT)/DCDC_thermische_Modellirung ==
  Diode_loss_kW : Inport
  igbt_loss_kW : Inport  Port=2
  "Heat sink Temperatur " : Constant  Value=DCT.thermal.heatsink_temperatur
  "Heat sink_Temperatur " : Constant  Value=DCT.thermal.heatsink_temperatur
  R_c_s_module_diode_side : Gain  Gain=DCT.thermal.R_c_s_module_diode_side
  R_c_s_module_igbt_side : Gain  Gain=DCT.thermal.R_c_s_module_igbt_side
  R_j_c_diode : Gain  Gain=DCT.thermal.R_j_c_diode
  R_j_c_igbt : Gain  Gain=DCT.thermal.R_j_c_igbt
  Sum : Sum  Inputs=|+++
  Sum1 : Sum  Inputs=|+++
  IGBT_Temp_Celsius : Outport
  Diode_Temp_Celsius : Outport  Port=2
  wires:
  igbt_loss_kW/1 -> R_j_c_igbt/1, R_c_s_module_igbt_side/1
  Diode_loss_kW/1 -> R_j_c_diode/1, R_c_s_module_diode_side/1
  "Heat sink Temperatur "/1 -> Sum/1
  "Heat sink_Temperatur "/1 -> Sum1/3
  R_j_c_diode/1 -> Sum1/2
  R_j_c_igbt/1 -> Sum/2
  R_c_s_module_igbt_side/1 -> Sum/3
  R_c_s_module_diode_side/1 -> Sum1/1
  Sum/1 -> IGBT_Temp_Celsius/1
  Sum1/1 -> Diode_Temp_Celsius/1

== system xEMU_SimulationModel3_rule1/Drive Train (DRT)/Aufteilung rad-undmotormomente ==
  F_EMAdemand_N : Inport
  F_brake_N : Inport  Port=2
  "WheelSpeed_rad/s " : Inport  Port=3
  Constant : Constant  Value=3
  Divide1 : Product  Inputs=*/
  Divide2 : Product  Inputs=/*
  Gain : Gain  Gain=gearratio_drt*60/2/pi
  Gain1 : Gain  Gain=R_wheel_drt_m/gearratio_drt
  Gain2 : Gain  Gain=R_wheel_drt_m
  T_demandperdrive_Nm : Outport
  n_motor_rpm : Outport  Port=2
  Number_drives_available : Outport  Port=3
  T_brake_axis_Nm : Outport  Port=4
  tag scope: num_EM=global
  wires:
  F_brake_N/1 -> Gain2/1
  Gain/1 -> n_motor_rpm/1
  Gain1/1 -> Divide1/1
  Constant/1 -> [num_EM], Divide2/1, Divide1/2, Number_drives_available/1
  Divide1/1 -> T_demandperdrive_Nm/1
  "WheelSpeed_rad/s "/1 -> Gain/1
  Gain2/1 -> Divide2/2
  Divide2/1 -> T_brake_axis_Nm/1
  F_EMAdemand_N/1 -> Gain1/1

== system xEMU_SimulationModel3_rule1/Drive Train (DRT)/Converter and traction motor ==
  T_demand : Inport
  n : Inport  Port=2
  v_dc : Inport  Port=3
  Converter_DRT : Subsystem
  Efficiency measument2 : Display
  Efficiency measurment1 : Subsystem
  Efficiency2 : Display
  Gain : Gain  Gain=2*pi/60
  Multiply : Product
  P_el : Display
  P_mech : Display
  Sum : Sum  Inputs=|++
  traction_motor_kennfeldbasiert : Subsystem
  "T_singelmotor_Nm " : Outport
  "Pel_singlemotor_kW " : Outport  Port=2
  tag scope: P_motor=global, Pv_ACDC=global, Pv_motor=global
  wires:
  Converter_DRT/2(Efficiency_out) -> Efficiency measument2/1
  traction_motor_kennfeldbasiert/1(P_el) -> P_el/1, [P_motor], Efficiency measurment1/1(In1), Sum/1
  v_dc/1 -> Converter_DRT/2(V_dcLinkStorage_V)
  Multiply/1 -> Gain/1
  Sum/1 -> "Pel_singlemotor_kW "/1
  n/1 -> Multiply/2, Converter_DRT/5(RPM), traction_motor_kennfeldbasiert/2(n)
  traction_motor_kennfeldbasiert/4(I_1) -> Converter_DRT/1("I_traction_motor ")
  traction_motor_kennfeldbasiert/2(M_ist) -> "T_singelmotor_Nm "/1
  Efficiency measurment1/1(Efficiency) -> Efficiency2/1
  traction_motor_kennfeldbasiert/3(U_1) -> Converter_DRT/3(V_Drive_V)
  traction_motor_kennfeldbasiert/6(Pv_motor) -> [Pv_motor]
  traction_motor_kennfeldbasiert/5(cos_phi) -> Converter_DRT/4(Cos_Phi_Phaseshift)
  T_demand/1 -> Multiply/1, traction_motor_kennfeldbasiert/1(M_soll)
  Converter_DRT/1(P_dcLinkTractionLoss_kW) -> Sum/2, Efficiency measurment1/2(In2), [Pv_ACDC]
  Gain/1 -> P_mech/1

== system xEMU_SimulationModel3_rule1/Drive Train (DRT)/Mechanical Brake ==
  In1 : Inport
  Out1 : Outport
  wires:
  In1/1 -> Out1/1

== system xEMU_SimulationModel3_rule1/Drive Train (DRT)/Slipmodel and Traction  ==
  T_EMAdemandper_axis_Nm : Inport
  v_train_m/s : Inport  Port=2
  adhesionCoefficient_abs : Inport  Port=3
  total mass_kg : Inport  Port=4
  numberdrivesavailable : Inport  Port=5
  "Tire Resistance " : Subsystem
  Variant Subsystem1 : Subsystem  Variant=on  OverrideUsingVariant=Variant2
  F_traction_peraxis_N : Outport
  WheelSpeed_rad/s : Outport  Port=2
  wires:
  "Tire Resistance "/1(resistance of tire) -> Variant Subsystem1/4(Resistance of tire)
  total mass_kg/1 -> "Tire Resistance "/2(total mass_kg)
  numberdrivesavailable/1 -> "Tire Resistance "/1(numberdrivesavailable)
  T_EMAdemandper_axis_Nm/1 -> Variant Subsystem1/1(T_EMAdemandper_axis_Nm)
  v_train_m/s/1 -> Variant Subsystem1/2(v_train_m/s)
  adhesionCoefficient_abs/1 -> Variant Subsystem1/3(adhesionCoefficient_abs)
  "Tire Resistance "/2(Fz_tire) -> Variant Subsystem1/5(Fz_tire)
  Variant Subsystem1/3(f_traction_tire) -> "Tire Resistance "/3(f_traction_tire)
  Variant Subsystem1/1(F_traction_peraxis_N) -> F_traction_peraxis_N/1
  Variant Subsystem1/2(WheelSpeed_rad/s) -> WheelSpeed_rad/s/1

== system xEMU_SimulationModel3_rule1/Energy Manager (EMA)/Berechnung der available Traktionsleitung ==
  P_load_available : Inport
  <P_motor_Verlust+Pacdc> : Inport  Port=2
  <P_dcdc_Verlust> : Inport  Port=3
  Subtract1 : Sum  Inputs=+-
  Subtract2 : Sum  Inputs=-+-
  Subtract3 : Sum  Inputs=+-
  eta_getriebe 1 : Gain
  P_traction_available : Outport
  wires:
  <P_dcdc_Verlust>/1 -> Subtract1/2
  <P_motor_Verlust+Pacdc>/1 -> Subtract3/2
  eta_getriebe 1/1 -> P_traction_available/1
  [P_clima] -> Subtract2/1
  [P_apu] -> Subtract2/3
  P_load_available/1 -> Subtract1/1
  Subtract3/1 -> eta_getriebe 1/1
  Subtract2/1 -> Subtract3/1
  Subtract1/1 -> Subtract2/2

== system xEMU_SimulationModel3_rule1/Energy Manager (EMA)/Kern von EMS ==
  note: P_load_wunsch_kw
  note: P_fc_kann
  P_load_wunsch_kw : Inport
  <v_train_m/s>_soll : Inport  Port=2
  <SOC_perc> : Inport  Port=3
  <V_bat_V> : Inport  Port=4
  Add : Sum
  Gain3 : Gain  Gain=1/100
  "Leistungsflussverteilug " : Subsystem
  P_load_aver : Subsystem
  Rate Limiter : RateLimiter  RisingSlewLimit=EMS.Fuelcell.P_fc_anstieg_max  FallingSlewLimit=EMS.Fuelcell.P_fc_abstieg_max  SampleTimeMode=inherited
  Saturation : Saturate  UpperLimit=EMS.Bat.power_discharge_max+EMS.Fuelcell.P_fc_max  LowerLimit=-EMS.Bat.power_charge_max + EMS.pload_average
  Saturation1 : Saturate  UpperLimit=EMS.Fuelcell.P_fc_max  LowerLimit=EMS.Fuelcell.P_fc_min
  Scope{1..4} (4 alike) : Scope
  Subsystem : Subsystem
  P_FCdemand_kW : Outport
  P_load_available : Outport  Port=2
  wires:
  <SOC_perc>/1 -> Gain3/1
  P_load_wunsch_kw/1 -> Saturation/1
  <v_train_m/s>_soll/1 -> P_load_aver/1(V_SOLL)
  Saturation/1 -> "Leistungsflussverteilug "/1(P_load), Subsystem/1(P_load_wunsch_kw), Scope2/1
  Gain3/1 -> P_load_aver/2(SOC), "Leistungsflussverteilug "/3(SoC), Subsystem/3(SOC)
  Add/1 -> P_load_available/1
  <V_bat_V>/1 -> Subsystem/4(<V_bat_V>)
  Subsystem/1(P_bat_kann) -> Add/2
  P_load_aver/1(P_load_mean) -> Scope3/1, "Leistungsflussverteilug "/2("P_load_aver ")
  Rate Limiter/1 -> Scope4/1, P_FCdemand_kW/1, Subsystem/2(P_fc_kann), Add/1
  Saturation1/1 -> Rate Limiter/1
  "Leistungsflussverteilug "/1(P_FCdemand_kW) -> Scope1/1, Saturation1/1

== system xEMU_SimulationModel3_rule1/Energy Manager (EMA)/Umrechnung von Kraft zu Leistung ==
  F_tractionDemand_N : Inport
  <v_train_m/s> : Inport  Port=2
  <P_motor_Verlust+Pacdc> : Inport  Port=3
  <P_dcdc_Verlust> : Inport  Port=4
  Constant2 : Constant  Value=10^-5
  Gain : Gain  Gain=1/ 1000
  Gain1 : Gain  Gain=1/ 1000
  Leistung nach ACDC : Sum
  Leistungsbedarf der Energiequelle : Sum
  Min2 : MinMax  Function=max  Inputs=2
  Product : Product
  Product1 : Product
  Sum1 : Sum  Inputs=|++
  "eta_getriebe " : Gain
  power into inverter1 : Sum  Inputs=+++
  P_load_wunsch : Outport
  P_drive_demand : Outport  Port=2
  tag scope: F_demand=global, F_driver=global
  wires:
  [F_EMA_min] -> Min2/2
  Min2/1 -> Product/1, [F_demand]
  Product/1 -> Gain/1
  Gain1/1 -> P_drive_demand/1  "P_drive_demand"
  Product1/1 -> Gain1/1
  F_tractionDemand_N/1 -> [F_driver], Product1/1, Min2/1
  "eta_getriebe "/1 -> Leistung nach ACDC/1  "P_drive_demand"
  Constant2/1 -> Sum1/2
  Sum1/1 -> Product/2
  Gain/1 -> "eta_getriebe "/1
  [P_apu] -> power into inverter1/3
  Leistungsbedarf der Energiequelle/1 -> P_load_wunsch/1  "P_load_wunsch"
  [P_clima] -> power into inverter1/2
  power into inverter1/1 -> Leistungsbedarf der Energiequelle/1
  Leistung nach ACDC/1 -> power into inverter1/1
  <P_motor_Verlust+Pacdc>/1 -> Leistung nach ACDC/2
  <P_dcdc_Verlust>/1 -> Leistungsbedarf der Energiequelle/2
  <v_train_m/s>/1 -> Sum1/1, Product1/2

== system xEMU_SimulationModel3_rule1/Energy Manager (EMA)/Umrechnung von Leistung auf Kraft ==
  P_traction_available : Inport
  P_drive_demand : Inport  Port=2
  <v_drivingCycle_m/s> : Inport  Port=3
  Constant3 : Constant  Value=10^-5
  Divide3 : Product  Inputs=*/
  Gain1 : Gain  Gain=1000
  Gain2 : Gain  Gain=1000
  MATLAB Function : MATLAB Function  TreatAsAtomicUnit=on
  MATLAB Function1 : MATLAB Function  TreatAsAtomicUnit=on
  MATLAB Function2 : MATLAB Function  TreatAsAtomicUnit=on
  Sum2 : Sum  Inputs=|++
  F_brakeMech_N : Outport
  F_EMAdemand_N : Outport  Port=2
  wires:
  MATLAB Function/1(y) -> Divide3/1
  P_traction_available/1 -> MATLAB Function2/2(P_tractionDemand)
  MATLAB Function2/1(P_EMAdemand) -> MATLAB Function1/1(u1)
  Constant3/1 -> Sum2/2
  Sum2/1 -> Divide3/2, MATLAB Function1/2(u2)
  Gain2/1 -> F_brakeMech_N/1
  P_drive_demand/1 -> MATLAB Function2/1(P_wunsch)
  Gain1/1 -> F_EMAdemand_N/1
  MATLAB Function2/2(P_brakeMech) -> MATLAB Function/1(u)
  MATLAB Function1/1(y) -> Gain1/1
  Divide3/1 -> Gain2/1
  <v_drivingCycle_m/s>/1 -> Sum2/1

== system xEMU_SimulationModel3_rule1/Energy Manager (EMA)/Umrechnung von Leistung auf Kraft2 ==
  F_brakeMech_N1 : Inport
  F_EMAdemand_N1 : Inport  Port=2
  <v_train_m/s> : Inport  Port=3
  Add : Sum
  MATLAB Function1 : MATLAB Function  TreatAsAtomicUnit=on
  F_available_nach_EMA : Outport
  F_brakeMech_N : Outport  Port=2
  F_EMAdemand_N : Outport  Port=3
  wires:
  MATLAB Function1/1(F_motor_nach_EMS) -> F_EMAdemand_N/1, Add/2
  F_brakeMech_N1/1 -> MATLAB Function1/6(F_brake_M_durch_P)
  [F_driver] -> MATLAB Function1/5(F_driver)
  [v_soll] -> MATLAB Function1/3(v_soll)
  MATLAB Function1/2(F_mech_nach_EMS) -> F_brakeMech_N/1, Add/1
  Add/1 -> F_available_nach_EMA/1  "F_available_nach_EMA"
  [F_demand] -> MATLAB Function1/4(F_motor_direkt)
  F_EMAdemand_N1/1 -> MATLAB Function1/1(F_motor_durch_P)
  <v_train_m/s>/1 -> MATLAB Function1/2(v)

== system xEMU_SimulationModel3_rule1/Fuel Cell System (FCS)/FC_DCDC  ==
  i_demand_ext : Inport
  V_dcLink : Inport  Port=2
  V_FCS : Inport  Port=3
  i_act_fcs : Inport  Port=4
  Product1 : Product
  Terminator : Terminator
  P_DCDC_act_kW : Outport
  i_demand_dcdc_fc : Outport  Port=2
  wires:
  Product1/1 -> P_DCDC_act_kW/1
  V_FCS/1 -> Product1/1
  i_act_fcs/1 -> Product1/2
  V_dcLink/1 -> Terminator/1
  i_demand_ext/1 -> i_demand_dcdc_fc/1
